simulink model "joint_space_adaptive"  (R2020b)
settings: Solver=VariableStepAuto  StartTime=0.0  StopTime=10.0  RelTol=1e-3
undefined symbols (not defined in the file): KD, Ktheta, lambda
settings Model: Creator=simon  LastModifiedBy=simon

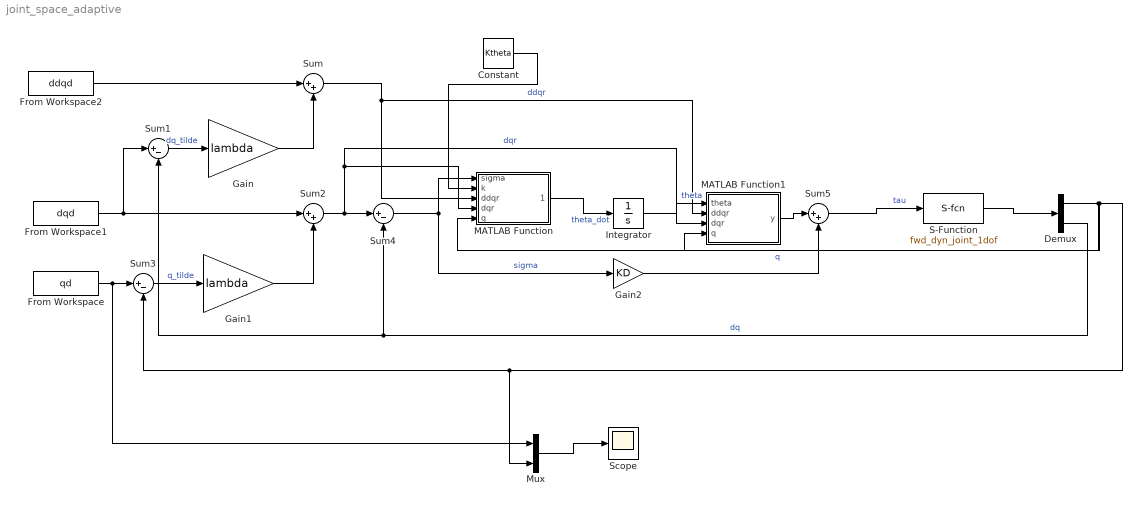
== system joint_space_adaptive ==
  Constant : Constant  Value=Ktheta
  Demux : Demux  Outputs=2
  From Workspace : FromWorkspace  VariableName=qd
  From Workspace1 : FromWorkspace  VariableName=dqd
  From Workspace2 : FromWorkspace  VariableName=ddqd
  Gain : Gain  Gain=lambda
  Gain1 : Gain  Gain=lambda
  Gain2 : Gain  Gain=KD
  Integrator : Integrator
  MATLAB Function : MATLAB Function  TreatAsAtomicUnit=on
  MATLAB Function1 : MATLAB Function  TreatAsAtomicUnit=on
  Mux : Mux  Inputs=2
  S-Function : S-Function  FunctionName=fwd_dyn_joint_1dof  Parameters=qi, dqi  SFunctionDeploymentMode=off  EnableBusSupport=off
  Scope : Scope
  Sum : Sum  Inputs=|++
  Sum1 : Sum  Inputs=|+-
  Sum2 : Sum  Inputs=|++
  Sum3 : Sum  Inputs=|+-
  Sum4 : Sum  Inputs=|+-
  Sum5 : Sum  Inputs=|++
  wires:
  From Workspace2/1 -> Sum/1
  Sum1/1 -> Gain/1  "dq_tilde"
  Gain/1 -> Sum/2
  From Workspace1/1 -> Sum2/1, Sum1/1
  Gain1/1 -> Sum2/2
  Sum3/1 -> Gain1/1  "q_tilde"
  From Workspace/1 -> Mux/1, Sum3/1
  Sum2/1 -> MATLAB Function1/3(dqr), MATLAB Function/4(dqr), Sum4/1  "dqr"
  Sum4/1 -> MATLAB Function/1(sigma), Gain2/1  "sigma"
  MATLAB Function/1(theta_dot) -> Integrator/1  "theta_dot"
  Integrator/1 -> MATLAB Function1/1(theta)  "theta"
  MATLAB Function1/1(y) -> Sum5/1
  S-Function/1 -> Demux/1
  Demux/1 -> MATLAB Function/5(q), MATLAB Function1/4(q), Mux/2, Sum3/2  "q"
  Demux/2 -> Sum1/2, Sum4/2  "dq"
  Gain2/1 -> Sum5/2
  Sum/1 -> MATLAB Function1/2(ddqr), MATLAB Function/3(ddqr)  "ddqr"
  Constant/1 -> MATLAB Function/2(k)
  Mux/1 -> Scope/1
  Sum5/1 -> S-Function/1  "tau"

== matlab function joint_space_adaptive/MATLAB Function1 ==
  data: theta input; y output; ddqr input; dqr input; q input
function y = fcn(theta, ddqr, dqr, q)

y = [ddqr dqr sin(q)]*theta;

== matlab function joint_space_adaptive/MATLAB Function ==
  data: sigma input; k input; theta_dot output size=3; ddqr input; dqr input; q input
function theta_dot = fcn(sigma,k,ddqr,dqr,q)

theta_dot = k*[ddqr;dqr;sin(q)];
